simulink model "SimulinkP8_1_Corrente"  (R2018b)
settings: Solver=VariableStepAuto  StartTime=0.0  StopTime=30  RelTol=1e-3
values from neighbouring files (symbols this model uses):
  C2 = [0 1]    [Problema8_1.m]
  Ca = [ 1 0; 0 1 ]    [Problema8_1.m]
  Da = [ 0; 0 ]    [Problema8_1.m]
  gama = [ 2; 1 ]    [Problema8_1.m]
  h = Wnh/Wn    [Problema8_1.m]
  L = [0 1] * inv(Wc)*(phi^2 + p1*phi + p2*eye(2))    [Problema8_1.m]
  Lc = ganho_dc/( C*inv( eye(2) - phi_cl )*gama )    [Problema8_1.m]
  phi = [1 Phi12; 0 0.4]    [Problema8_1.m]
  xobs = [0 0]'    [Problema8_1.m]    (also in corrente.m = (eye(2)-Ko*C)*phi*xobs + (eye(2)-Ko*C)*gama*uk + Ko*yk)
settings Model: Creator=root  LastModifiedBy=root

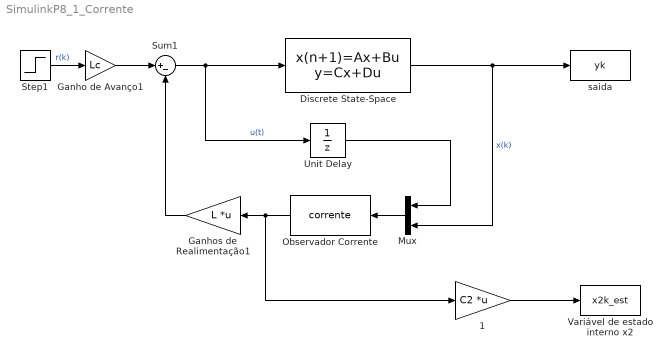
== system SimulinkP8_1_Corrente ==
  " saida" : ToWorkspace  VariableName=yk  SaveFormat=Structure With Time  SampleTime=-1
  1 : Gain  Gain=C2  Multiplication=Matrix(K*u) (u vector)
  Discrete State-Space : DiscreteStateSpace  A=phi  B=gama  C=Ca  D=Da  InitialCondition=xobs  SampleTime=h
  Ganho de Avanço1 : Gain  Gain=Lc
  Ganhos de Realimentação1 : Gain  Gain=L  Multiplication=Matrix(K*u) (u vector)
  Mux : Mux  Inputs=2
  Observador Corrente : MATLABFcn  MATLABFcn=corrente  OutputDimensions=2
  Step1 : Step  Time=0  SampleTime=0
  Sum1 : Sum  Inputs=|+-
  Unit Delay : UnitDelay  SampleTime=-1
  Variável de estado interno x2 : ToWorkspace  VariableName=x2k_est  SaveFormat=Structure With Time  SampleTime=-1
  wires:
  Mux/1 -> Observador Corrente/1
  Observador Corrente/1 -> 1/1, Ganhos de Realimentação1/1
  Ganhos de Realimentação1/1 -> Sum1/2
  Sum1/1 -> Unit Delay/1, Discrete State-Space/1  "u(t)"
  Discrete State-Space/1 -> Mux/2, " saida"/1  "x(k)"
  Step1/1 -> Ganho de Avanço1/1  "r(k)"
  Ganho de Avanço1/1 -> Sum1/1
  1/1 -> Variável de estado interno x2/1
  Unit Delay/1 -> Mux/1
